simulink model "EKFSim"  (R2012b)
settings: Solver=VariableStepDiscrete  SolverMode=SingleTasking  StartTime=0.0  StopTime=TFinal  FixedStep=Ts  MaxStep=Ts  RelTol=1e-3
values from neighbouring files (symbols this model uses):
  cx = 2    [EKFDriver.m]
  cy = 2    [EKFDriver.m]
  muWx = 0    [EKFDriver.m]
  muWy = 0    [EKFDriver.m]
  P0 = [1;1]    [EKFDriver.m]
  sigB = 1e-1    (= 0.1)    [EKFDriver.m]
  sigR = 1e-1    (= 0.1)    [EKFDriver.m]
  sigWx = 1e-7    (= 1e-07)    [EKFDriver.m]
  sigWy = 1e-7    (= 1e-07)    [EKFDriver.m]
  Ts = 1/100    (= 0.01)    [EKFDriver.m]
  V0 = [-0.25;0.25]    [EKFDriver.m]
  wx = 0    [EKFDriver.m]
  wy = 0    [EKFDriver.m]
  Z = 2    [EKFDriver.m]
undefined symbols (not defined in the file or in its folder): randraw
settings Model: SimulationMode=accelerator  Creator=sqn4594  LastModifiedBy=sqn4594
settings DataIOCC: SignalLoggingSaveFormat=ModelDataLogs  InspectSignalLogs=on
settings DebuggingCC: MultiTaskDSMMsg=warning  MultiTaskCondExecSysMsg=none  StrictBusMsg=None
settings HardwareCC: ProdBitPerInt=16  ProdBitPerPointer=8  ProdIntDivRoundTo=Zero  ProdEndianess=LittleEndian  ProdWordSize=8  ProdHWDeviceType=Atmel->AVR  TargetIntDivRoundTo=Zero  TargetEndianess=LittleEndian  TargetHWDeviceType=MATLAB Host  ProdEqTarget=off
settings SFSimCC: SimParseCustomCode=off
settings RTWCC: SystemTargetFile=rsim.tlc  TemplateMakefile=rsim_default_tmf  Description=Rapid Simulation Target  RTWVerbose=off  ProcessScript=rsim_make_rtw_hook  IncludeERTFirstTime=on
settings CodeAppCC: CustomSymbolStrType=$N$R$M_T  InternalIdentifier=Shortened
settings RSimTargetCC: CodeReplacementLibrary=ANSI_C  ERTMultiwordTypeDef=System defined  ERTMultiwordLength=256  IsPILTarget=off  EnableShiftOperators=on

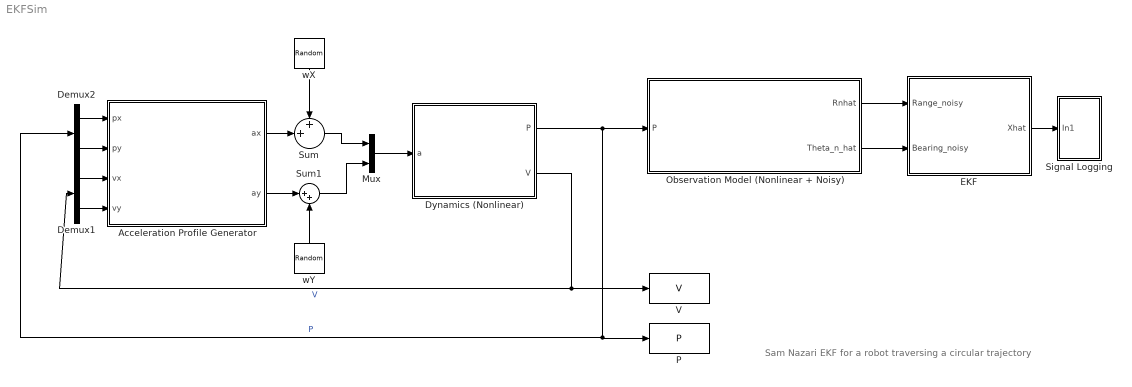
== system EKFSim ==
  note: Sam Nazari
      | EKF for a robot traversing a circular trajectory
  Acceleration Profile Generator : Subsystem
  Demux1 : Demux  Outputs=2
  Demux2 : Demux  Outputs=2
  Dynamics (Nonlinear) : Subsystem
  EKF : Subsystem
  Mux : Mux  Inputs=2
  Observation Model (Nonlinear + Noisy) : Subsystem
  "P " : ToWorkspace  VariableName=P  SampleTime=-1
  Signal Logging : Subsystem
  Sum : Sum  Inputs=++|
  Sum1 : Sum  Inputs=|++
  "V " : ToWorkspace  VariableName=V  SampleTime=-1
  wX : RandomNumber  Mean=muWx  Variance=sigWx  Seed=2^wx  SampleTime=Ts
  wY : RandomNumber  Mean=muWy  Variance=sigWy  Seed=2^wy  SampleTime=Ts
  wires:
  Acceleration Profile Generator/1(ax) -> Sum/2
  Acceleration Profile Generator/2(ay) -> Sum1/1
  Sum/1 -> Mux/1
  Sum1/1 -> Mux/2
  Demux1/1 -> Acceleration Profile Generator/3(vx)
  Demux1/2 -> Acceleration Profile Generator/4(vy)
  wX/1 -> Sum/1
  wY/1 -> Sum1/2
  Demux2/1 -> Acceleration Profile Generator/1(px)
  Demux2/2 -> Acceleration Profile Generator/2(py)
  Dynamics (Nonlinear)/1("P ") -> "P "/1, Demux2/1, Observation Model (Nonlinear + Noisy)/1("P ")  "P"
  Mux/1 -> Dynamics (Nonlinear)/1(a)
  Dynamics (Nonlinear)/2("V ") -> "V "/1, Demux1/1  "V"
  Observation Model (Nonlinear + Noisy)/1("Rnhat ") -> EKF/1(Range_noisy)
  Observation Model (Nonlinear + Noisy)/2("Theta_n_hat ") -> EKF/2(Bearing_noisy)
  EKF/1(Xhat) -> Signal Logging/1(In1)

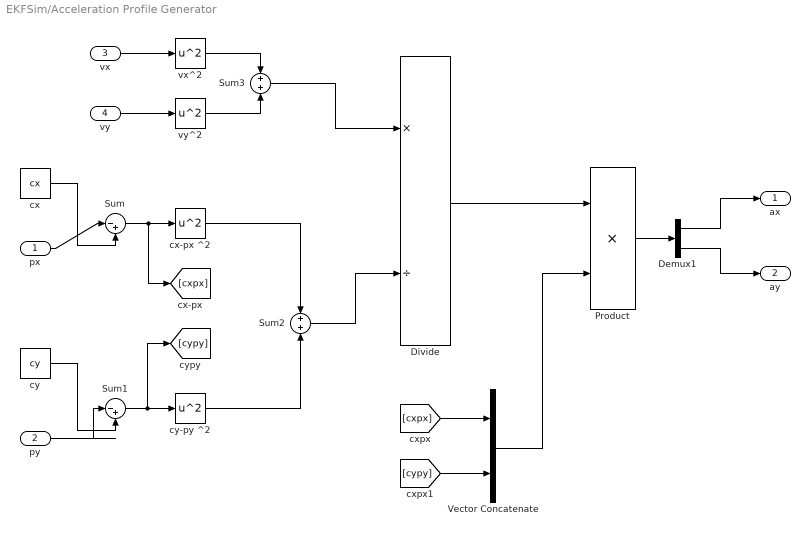
== system EKFSim/Acceleration Profile Generator ==
  px : Inport
  py : Inport  Port=2
  vx : Inport  Port=3
  vy : Inport  Port=4
  Demux1 : Demux  Outputs=2
  Divide : Product  Inputs=*/
  Product : Product
  Sum : Sum  Inputs=|-+
  Sum1 : Sum  Inputs=|-+
  Sum2 : Sum
  Sum3 : Sum
  Vector Concatenate : Concatenate  ConcatenateDimension=2
  cx : Constant  Value=cx
  cx-px ^2 : Math  Operator=square  SaturateOnIntegerOverflow=on
  cy : Constant  Value=cy
  cy-py ^2 : Math  Operator=square  SaturateOnIntegerOverflow=on
  vx^2 : Math  Operator=square  SaturateOnIntegerOverflow=on
  vy^2 : Math  Operator=square  SaturateOnIntegerOverflow=on
  ax : Outport
  ay : Outport  Port=2
  wires:
  Sum3/1 -> Divide/1
  vy^2/1 -> Sum3/2
  cy/1 -> Sum1/2
  vy/1 -> vy^2/1
  [cxpx] -> Vector Concatenate/1
  cx/1 -> Sum/2
  px/1 -> Sum/1
  vx/1 -> vx^2/1
  Sum/1 -> [cxpx], cx-px ^2/1
  Sum1/1 -> [cypy], cy-py ^2/1
  cy-py ^2/1 -> Sum2/2
  cx-px ^2/1 -> Sum2/1
  Divide/1 -> Product/1
  vx^2/1 -> Sum3/1
  [cypy] -> Vector Concatenate/2
  Vector Concatenate/1 -> Product/2
  Demux1/1 -> ax/1
  Sum2/1 -> Divide/2
  Product/1 -> Demux1/1
  Demux1/2 -> ay/1
  py/1 -> Sum1/1

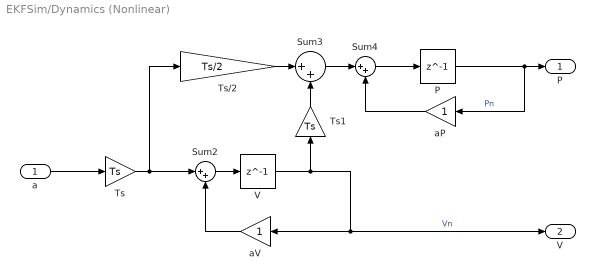
== system EKFSim/Dynamics (Nonlinear) ==
  a : Inport
  P : Delay  DelayLength=1  InitialCondition=P0
  Sum2 : Sum  Inputs=|++
  Sum3 : Sum  Inputs=|++
  Sum4 : Sum  Inputs=|++
  Ts : Gain  Gain=Ts
  Ts/2 : Gain  Gain=Ts/2
  Ts1 : Gain  Gain=Ts
  V : Delay  DelayLength=1  InitialCondition=V0
  aP : Gain
  aV : Gain
  "P " : Outport
  "V " : Outport  Port=2
  wires:
  V/1 -> "V "/1, aV/1, Ts1/1  "Vn"
  Sum2/1 -> V/1
  aV/1 -> Sum2/2
  a/1 -> Ts/1
  P/1 -> "P "/1, aP/1  "Pn"
  Ts/1 -> Ts/2/1, Sum2/1
  Ts1/1 -> Sum3/2
  Sum3/1 -> Sum4/1
  aP/1 -> Sum4/2
  Ts/2/1 -> Sum3/1
  Sum4/1 -> P/1

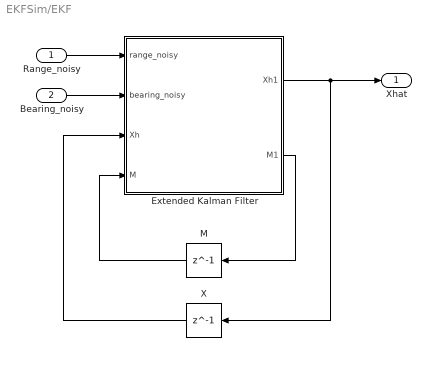
== system EKFSim/EKF ==
  Range_noisy : Inport
  Bearing_noisy : Inport  Port=2
  Extended Kalman Filter : MATLAB Function  TreatAsAtomicUnit=on
  M : Delay  DelayLength=1  InitialCondition=zeros(4,4)
  X : Delay  DelayLength=1  InitialCondition=[P0;V0]
  Xhat : Outport
  wires:
  Extended Kalman Filter/1(Xh1) -> Xhat/1, X/1
  Range_noisy/1 -> Extended Kalman Filter/1(range_noisy)
  Bearing_noisy/1 -> Extended Kalman Filter/2(bearing_noisy)
  M/1 -> Extended Kalman Filter/4(M)
  Extended Kalman Filter/2(M1) -> M/1
  X/1 -> Extended Kalman Filter/3(Xh)

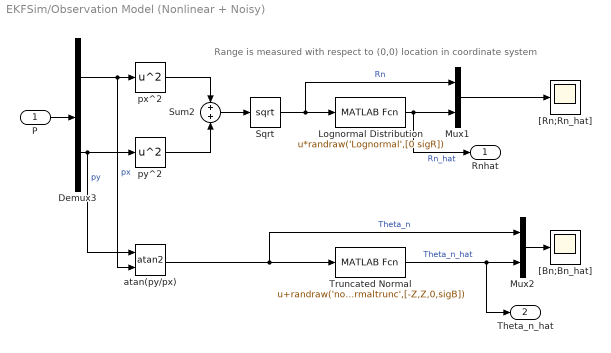
== system EKFSim/Observation Model (Nonlinear + Noisy) ==
  note: Range is measured with respect to (0,0) location in coordinate system
  "P " : Inport
  Demux3 : Demux  Outputs=2
  Lognormal Distribution : MATLABFcn  MATLABFcn=u*randraw('Lognormal',[0 sigR])
  Mux1 : Mux  Inputs=2
  Mux2 : Mux  Inputs=2
  Sqrt : Sqrt  SaturateOnIntegerOverflow=on
  Sum2 : Sum
  Truncated Normal : MATLABFcn  MATLABFcn=u+randraw('normaltrunc',[-Z,Z,0,sigB])
  "[Bn;Bn_hat]" : Scope
      settings: SaveName=Bnhat
  "[Rn;Rn_hat]" : Scope
      settings: SaveName=Rnhat
  atan(py/px) : Trigonometry  Operator=atan2
  px^2 : Math  Operator=square  SaturateOnIntegerOverflow=on
  py^2 : Math  Operator=square  SaturateOnIntegerOverflow=on
  "Rnhat " : Outport
  "Theta_n_hat " : Outport  Port=2
  wires:
  Mux1/1 -> "[Rn;Rn_hat]"/1
  atan(py/px)/1 -> Mux2/1, Truncated Normal/1  "Theta_n"
  Mux2/1 -> "[Bn;Bn_hat]"/1
  "P "/1 -> Demux3/1
  Sum2/1 -> Sqrt/1
  px^2/1 -> Sum2/1
  py^2/1 -> Sum2/2
  Sqrt/1 -> Mux1/1, Lognormal Distribution/1  "Rn"
  Demux3/2 -> atan(py/px)/1, py^2/1  "py"
  Demux3/1 -> atan(py/px)/2, px^2/1  "px"
  Truncated Normal/1 -> "Theta_n_hat "/1, Mux2/2  "Theta_n_hat"
  Lognormal Distribution/1 -> "Rnhat "/1, Mux1/2  "Rn_hat"

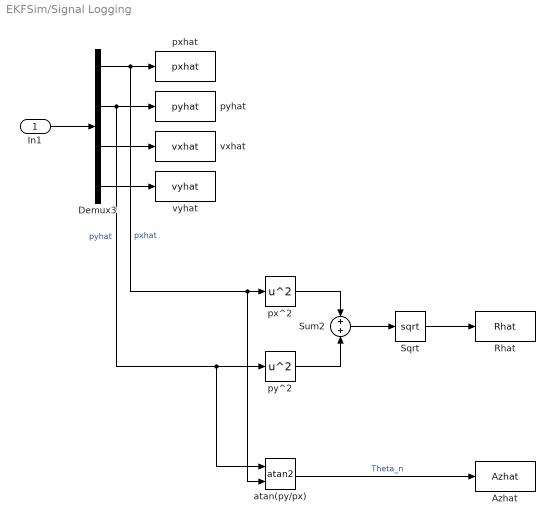
== system EKFSim/Signal Logging ==
  In1 : Inport
  "Azhat " : ToWorkspace  VariableName=Azhat  SampleTime=-1
  Demux3 : Demux
  Rhat : ToWorkspace  VariableName=Rhat  SampleTime=-1
  Sqrt : Sqrt  SaturateOnIntegerOverflow=on
  Sum2 : Sum
  atan(py/px) : Trigonometry  Operator=atan2
  px^2 : Math  Operator=square  SaturateOnIntegerOverflow=on
  pxhat : ToWorkspace  VariableName=pxhat  SampleTime=-1
  py^2 : Math  Operator=square  SaturateOnIntegerOverflow=on
  pyhat : ToWorkspace  VariableName=pyhat  SampleTime=-1
  vxhat : ToWorkspace  VariableName=vxhat  SampleTime=-1
  vyhat : ToWorkspace  VariableName=vyhat  SampleTime=-1
  wires:
  In1/1 -> Demux3/1
  Demux3/3 -> vxhat/1
  Demux3/4 -> vyhat/1
  px^2/1 -> Sum2/1
  py^2/1 -> Sum2/2
  Demux3/2 -> atan(py/px)/1, py^2/1, pyhat/1  "pyhat"
  Demux3/1 -> atan(py/px)/2, px^2/1, pxhat/1  "pxhat"
  atan(py/px)/1 -> "Azhat "/1  "Theta_n"
  Sum2/1 -> Sqrt/1
  Sqrt/1 -> Rhat/1

== matlab function EKFSim/EKF/Extended Kalman Filter ==
  data: range_noisy input; bearing_noisy input; Xh input; M input; Xh1 output; M1 output
function [Xh1,M1] = EKF(range_noisy,bearing_noisy,Xh,M)
%#codegen
Ts = 1/100;

sigWx   = 2e-9;
sigWy   = 1e-9;

sigR    = 1e-2;
sigB    = 1e-2;

% Form Q
Q       = [sigWx 0;0 sigWy];
R       = [sigR 0; 0 sigB];

cx      = 2;
cy      = 2;

px      = Xh(1);
py      = Xh(2);
vx      = Xh(3);
vy      = Xh(4);


%% Compute partials for Update...

%F
a = (cx-px)^2+(cy-py)^2;
b = vx^2+vy^2;
c = b/a;

f11 = 1+c*((cx-px)^2/a -(1/2))*Ts^2;
f12 = c*(1/a)*(cx-px)*(cy-py)*Ts^2;
f13 = (1/a)*vx*(cx-px)*Ts^2;
f14 = (1/a)*vy*(cy-py)*Ts^2;

f21 = c*(1/a)*(cx-px)*(cy-py)*Ts^2;
f22 = 1+(Ts^2*c*((1/a)*(cy-py)^2 - (1/2)));
f23 = (Ts/a)*(vx*(cy-py));
f24 = Ts+((vy/a)*(cy-py))*Ts^2;

f31 = c*(Ts*(2/a)*(cx-px)^2-Ts);
f32 = (2*Ts*c)*(1/a)*(cy-py)*(cx-px);
f33 = 1+(2*Ts/a)*vx*(cx-px);
f34 = (2*Ts/a)*vy*(cx-px);

f41 = 2*(c/a)*(cx-px)*(cy-py);
f42 = c*((2/a)*(cy-py)^2 - 1)*Ts;
f43 = (2*Ts/a)*vx*(cy-py);
f44 = 1+(2*Ts/a)*(cy-py);

F = [f11 f12 f13 f14;
    f21 f22 f23 f24;
    f31 f32 f33 f34;
    f41 f42 f43 f44];

%L
l11 = (Ts^2)/2;
l12 = 0;
l21 = 0;
l22 = l11;
l31 = Ts;
l32 = 0;
l41 = 0;
l42 = Ts;

L = [l11 l12; l21 l22; l31 l32; l41 l42];

%% Time Update of State & Covariance
P = [px;py];
V = [vx;vy];

X = [P;V];

ax = ((vx^2 + vy^2)*(cx - px))/((cx - px)^2 + (cy - py)^2);
ay = ((vx^2 + vy^2)*(cy - py))/((cx - px)^2 + (cy - py)^2);

alph = [ax;ay];

fup = [P;zeros(2,1)]+[Ts*V;V]+Ts*[zeros(2,1);alph]+((Ts^2)/2)*[alph;zeros(2,1)];
Mup = F*M*F'+L*Q*L';

pxup = fup(1);
pyup = fup(2);
vxup = fup(3);
vyup = fup(4);

%% Compute Partials for Observation
H   = [            0                 0                0 0;
       -pyup/(pxup^2 + pyup^2),pxup/(pxup^2 + pyup^2),0,0];

Mk   = [(pxup^2 + pyup^2)^(1/2), 0;
         0,                   1];
     
%% Measurement update

K   = Mup*H'*inv(H*Mup*H'+Mk*R*Mk');
Xh1 = fup+K*([range_noisy;bearing_noisy]-[(pxup^2+pyup^2)^0.5;atan2(pyup,pxup)]);
M1  = (eye(4)-K*H)*Mup;
